simulink model "sim_control_old_version"  (Simulink 9.2)
settings: Solver=ode45  StartTime=0.0  StopTime=Tsim  FixedStep=0.001  MaxStep=1e-4  RelTol=1e-3  EnableMultiTasking=on
values from neighbouring files (symbols this model uses):
  c = 4    [call_sim.m]    (also in gm_pm.m = 10.9123)
  k = 400    [call_sim.m]    (also in gm_pm.m = 451.39)
  Kd = 0.1    [call_sim.m]    (also in gm_pm.m = 0)
  Ki = 8    [call_sim.m]    (also in gm_pm.m = 0)
  Kp = 3    [call_sim.m]    (also in gm_pm.m = 2000)
  m = 0.79    [call_sim.m]    (also in gm_pm.m = 0.8775)
  v0 = 0    [call_sim.m]
  x0 = 0    [call_sim.m]
settings Model: Creator=snahata  LastModifiedBy=akashgarg
settings OptimizationCC: InitFltsAndDblsToZero=on
settings DebuggingCC: SaveWithParameterizedLinksMsg=none  SignalResolutionControl=TryResolveAllWithWarning  SolverPrmCheckMsg=warning  MultiTaskDSMMsg=warning  MultiTaskCondExecSysMsg=none
settings GRTTargetCC: TargetFcnLib=ansi_tfl_tmw.mat

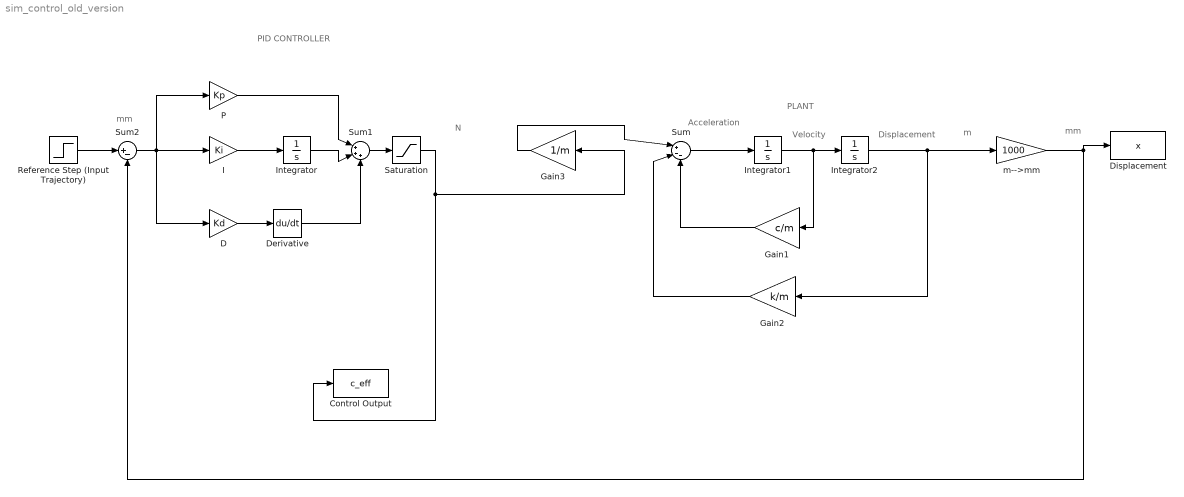
== system sim_control_old_version ==
  note: Acceleration
  note: Velocity
  note: Displacement
  note: mm
  note: N
  note: m
  note: mm
  note: PID CONTROLLER
  note: PLANT
  Control Output : ToWorkspace  VariableName=c_eff  SaveFormat=Timeseries  SampleTime=-1
  D : Gain  Gain=Kd
  Derivative : Derivative
  Displacement : ToWorkspace  VariableName=x  SaveFormat=Timeseries  SampleTime=-1
  Gain1 : Gain  Gain=c/m
  Gain2 : Gain  Gain=k/m
  Gain3 : Gain  Gain=1/m
  I : Gain  Gain=Ki
  Integrator : Integrator
  Integrator1 : Integrator  InitialCondition=v0
  Integrator2 : Integrator  InitialCondition=x0
  P : Gain  Gain=Kp
  Reference Step (Input Trajectory) : Step  After=3  SampleTime=0.01
  Saturation : Saturate  UpperLimit=15  LowerLimit=-15
  Sum : Sum  Inputs=|+--
  Sum1 : Sum  Inputs=|+++
  Sum2 : Sum  Inputs=|+-
  m-->mm : Gain  Gain=1000
  wires:
  Sum/1 -> Integrator1/1
  Integrator1/1 -> Integrator2/1, Gain1/1
  Gain1/1 -> Sum/3
  Gain2/1 -> Sum/2
  Integrator2/1 -> Gain2/1, m-->mm/1
  D/1 -> Derivative/1
  I/1 -> Integrator/1
  Integrator/1 -> Sum1/2
  Derivative/1 -> Sum1/3
  P/1 -> Sum1/1
  Sum1/1 -> Saturation/1
  Sum2/1 -> D/1, I/1, P/1
  m-->mm/1 -> Displacement/1, Sum2/2
  Reference Step (Input Trajectory)/1 -> Sum2/1
  Saturation/1 -> Control Output/1, Gain3/1
  Gain3/1 -> Sum/1
